simulink model "disturbed_pitch_system"  (R2019b)
settings: Solver=VariableStepAuto  StartTime=0.0  StopTime=4  RelTol=1e-3
undefined symbols (not defined in the file or in its folder): G_theta_samples
libraries: simulink x12, cstblocks x5
settings Model: Creator=amirhossein  LastModifiedBy=amirhossein

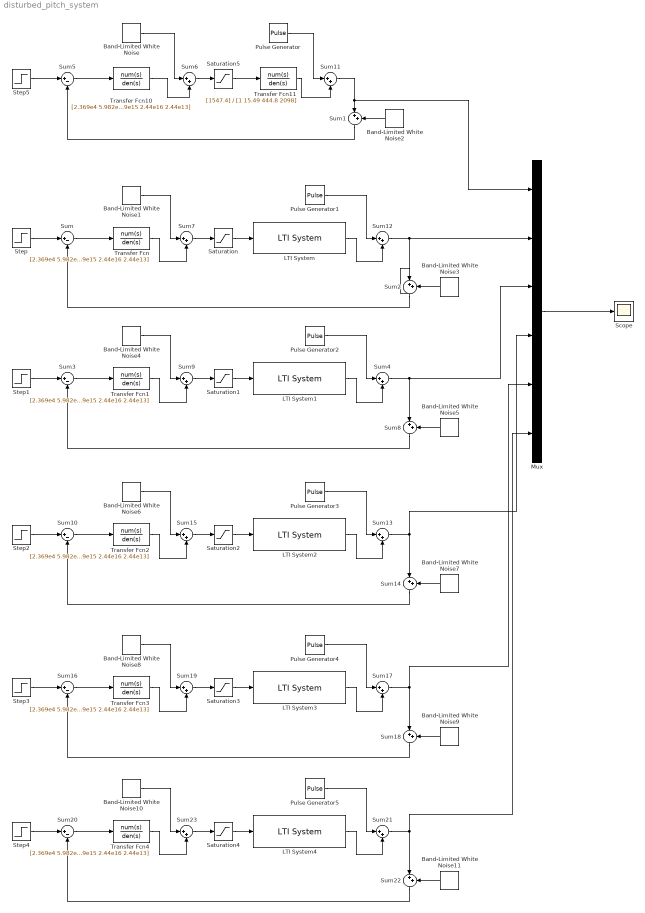
== system disturbed_pitch_system ==
  Band-Limited White Noise{,1,4,6,8,10} (6 alike) : simulink/Sources/Band-Limited White Noise  Cov=[0.001]  Ts=0.01  seed=[23341]
  Band-Limited White Noise{2..3,5,7,9,11} (6 alike) : simulink/Sources/Band-Limited White Noise  Cov=[0.0001]  Ts=0.01  seed=[23341]
  LTI System : cstblocks/LTI System  sys=G_theta_samples(: , : , 1)  IC=[]
  LTI System1 : cstblocks/LTI System  sys=G_theta_samples(: , : , 2)  IC=[]
  LTI System2 : cstblocks/LTI System  sys=G_theta_samples(: , : , 3)  IC=[]
  LTI System3 : cstblocks/LTI System  sys=G_theta_samples(: , : , 4)  IC=[]
  LTI System4 : cstblocks/LTI System  sys=G_theta_samples(: , : , 5)  IC=[]
  Mux : Mux  Inputs=6
  Pulse Generator{,1..5} (6 alike) : DiscretePulseGenerator  PulseType=Time based  Amplitude=0.1  Period=1.5  PulseWidth=5
  Saturation{,1..5} (6 alike) : Saturate  UpperLimit=20  LowerLimit=-20
  Scope : Scope
  Step{,1..5} (6 alike) : Step  SampleTime=0
  Sum{,3,5,10,16,20} (6 alike) : Sum  Inputs=|+-
  Sum{1..2,4,6..9,11..15,17..19,21..23} (18 alike) : Sum  Inputs=|++
  Transfer Fcn{,1..4,10} (6 alike) : TransferFcn  Numerator=[2.369e4 5.982e8 2.858e11 1.872e13 4.554e14 8.612e15 7.941e16 2.344e17]  Denominator=[1 2.715e4 6.056e7 3.819e10 3.997e12 2.165e14 4.539e15 2.44e16 2.44e13]
  Transfer Fcn11 : TransferFcn  Numerator=[1547.4]  Denominator=[1 15.49 444.8 2098]
  wires:
  Transfer Fcn/1 -> Sum7/2
  Saturation5/1 -> Transfer Fcn11/1
  Step/1 -> Sum/1
  Saturation/1 -> LTI System/1
  Sum5/1 -> Transfer Fcn10/1
  Sum/1 -> Transfer Fcn/1
  Step5/1 -> Sum5/1
  Transfer Fcn10/1 -> Sum6/2
  Band-Limited White Noise/1 -> Sum6/1
  Sum6/1 -> Saturation5/1
  Band-Limited White Noise1/1 -> Sum7/1
  Sum7/1 -> Saturation/1
  Pulse Generator/1 -> Sum11/1
  Transfer Fcn11/1 -> Sum11/2
  Sum1/1 -> Sum5/2
  Sum11/1 -> Sum1/1, Mux/1
  Band-Limited White Noise2/1 -> Sum1/2
  LTI System/1 -> Sum12/2
  Pulse Generator1/1 -> Sum12/1
  Band-Limited White Noise3/1 -> Sum2/2
  Sum12/1 -> Sum2/1, Mux/2
  Sum2/1 -> Sum/2
  Mux/1 -> Scope/1
  Transfer Fcn1/1 -> Sum9/2
  Step1/1 -> Sum3/1
  Saturation1/1 -> LTI System1/1
  Pulse Generator2/1 -> Sum4/1
  Sum8/1 -> Sum3/2
  Sum3/1 -> Transfer Fcn1/1
  Band-Limited White Noise4/1 -> Sum9/1
  Sum9/1 -> Saturation1/1
  Sum4/1 -> Mux/3, Sum8/1
  Band-Limited White Noise5/1 -> Sum8/2
  LTI System1/1 -> Sum4/2
  Pulse Generator3/1 -> Sum13/1
  Sum15/1 -> Saturation2/1
  LTI System2/1 -> Sum13/2
  Band-Limited White Noise7/1 -> Sum14/2
  Sum10/1 -> Transfer Fcn2/1
  Saturation2/1 -> LTI System2/1
  Sum14/1 -> Sum10/2
  Transfer Fcn2/1 -> Sum15/2
  Sum13/1 -> Mux/4, Sum14/1
  Band-Limited White Noise6/1 -> Sum15/1
  Step2/1 -> Sum10/1
  Sum18/1 -> Sum16/2
  Sum19/1 -> Saturation3/1
  Band-Limited White Noise8/1 -> Sum19/1
  Transfer Fcn3/1 -> Sum19/2
  LTI System3/1 -> Sum17/2
  Sum17/1 -> Mux/5, Sum18/1
  Sum16/1 -> Transfer Fcn3/1
  Step3/1 -> Sum16/1
  Pulse Generator4/1 -> Sum17/1
  Saturation3/1 -> LTI System3/1
  Band-Limited White Noise9/1 -> Sum18/2
  Sum21/1 -> Mux/6, Sum22/1
  Band-Limited White Noise11/1 -> Sum22/2
  Band-Limited White Noise10/1 -> Sum23/1
  LTI System4/1 -> Sum21/2
  Pulse Generator5/1 -> Sum21/1
  Saturation4/1 -> LTI System4/1
  Sum20/1 -> Transfer Fcn4/1
  Sum23/1 -> Saturation4/1
  Transfer Fcn4/1 -> Sum23/2
  Step4/1 -> Sum20/1
  Sum22/1 -> Sum20/2
